simulink model "TEST_Parsim"  (R2020b)
settings: Solver=VariableStepAuto  StartTime=0.0  StopTime=10.0  RelTol=1e-3
undefined symbols (not defined in the file or in its folder): TEST_PARSIM
settings Model: Creator=sl  LastModifiedBy=sl

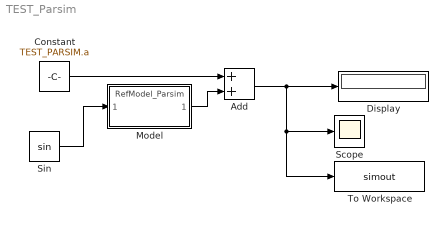
== system TEST_Parsim ==
  Add : Sum
  Constant : Constant  Value=TEST_PARSIM.a
  Display : Display
  Model : ModelReference  ModelNameDialog=RefModel_Parsim.slx  SimulationMode=Normal  ModelReferenceVersion=1.1
  Scope : Scope
  Sin : Trigonometry
  To Workspace : ToWorkspace  VariableName=simout  SaveFormat=Timeseries  SampleTime=-1
  wires:
  Constant/1 -> Add/1
  Sin/1 -> Model/1
  Add/1 -> To Workspace/1, Scope/1, Display/1
  Model/1 -> Add/2
